simulink model "sampleModel1898"  (R2023a)
settings: Solver=VariableStepAuto  StartTime=0.0  StopTime=10.0  RelTol=1e-3
libraries: simulink x5, hdlsllib x3
settings Model: Creator=user1  LastModifiedBy=user1

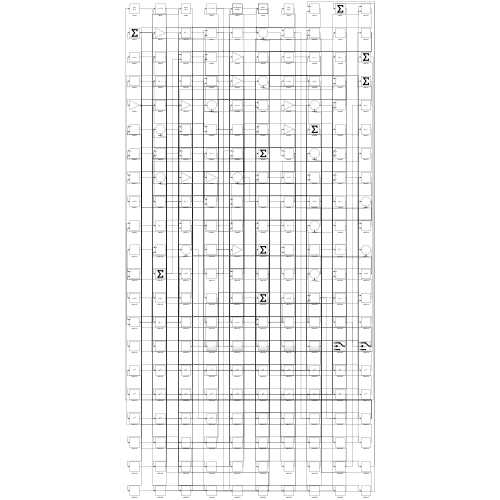
[thumbnail: Simulink's stored preview of the top-level diagram]
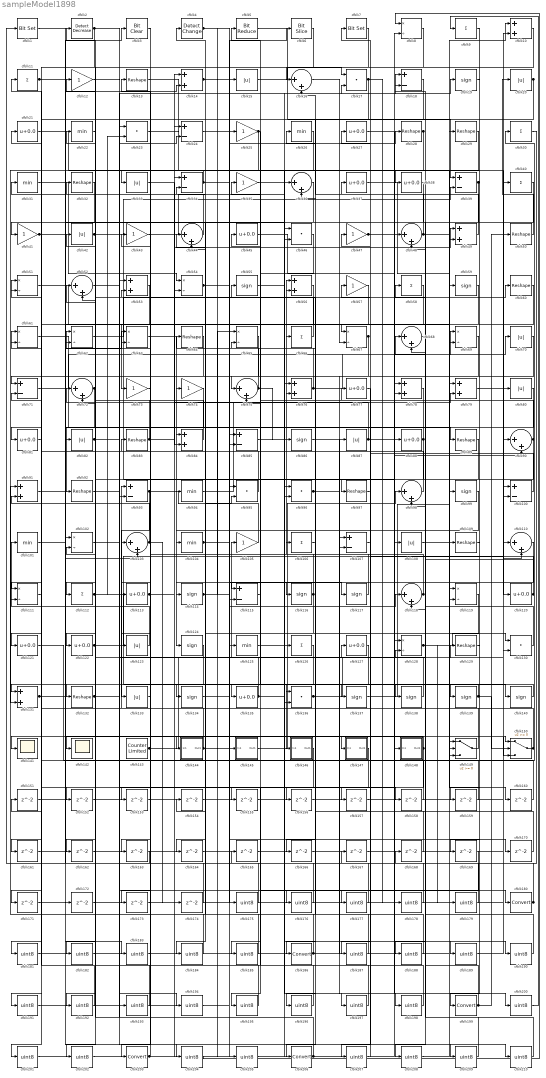
== system sampleModel1898 ==
  cfblk1 : simulink/Logic and Bit Operations/Bit Set  iBit=0
      settings: LibrarySourceBlock=|
      | hdlsllib/Logic and Bit
      | Operations/Bit Set
  cfblk{10,14,49,53,56,76,78..79,84,91,131} (11 alike) : Sum
  cfblk{18,24,34,39,71,85,93,100,107,115} (10 alike) : Sum  Inputs=+-
  cfblk{22,26,31,94,101,104,125} (7 alike) : MinMax
  cfblk{8,51,54,61..63,65,67,69,102,111,119,128} (13 alike) : Product  Inputs=*/  RndMeth=Zero  SaturateOnIntegerOverflow=on
  cfblk{16,36,44,48,52,68,72,75,90,98,103,110,118} (13 alike) : Sum  Inputs=|++
  cfblk{12,25,35,41,43,47,57,73..74,105} (10 alike) : Gain
  cfblk{9,11,30,40,58,66,106,112,126} (9 alike) : Sum  Inputs=+
  cfblk{15,20,33,42,70,80,82,87,108,123,133} (11 alike) : Abs  SaturateOnIntegerOverflow=off
  cfblk{13,28..29,32,50,60,64,83,89,92,97,109,129,132} (14 alike) : Reshape
  cfblk{21,27,37..38,45,77,81,88,113,120..122,127,135} (14 alike) : Bias  Bias=0.0  SaturateOnIntegerOverflow=off
  cfblk{19,55,59,86,99,114,116..117,124,134,137..140} (14 alike) : Signum
  cfblk{17,23,46,95..96,130,136} (7 alike) : DotProduct  OutDataTypeStr=Inherit: Inherit via internal rule
  cfblk141 : Scope
  cfblk142 : Scope
  cfblk143 : hdlsllib/Sources/Counter Limited  uplimit=7  tsamp=-1
  cfblk144 : Subsystem
      settings: LibrarySourceBlock=|
      | hdlsllib/Ports &
      | Subsystems/Subsystem
  cfblk145 : Subsystem
      settings: LibrarySourceBlock=|
      | hdlsllib/Ports &
      | Subsystems/Subsystem
  cfblk146 : Subsystem
      settings: LibrarySourceBlock=|
      | hdlsllib/Ports &
      | Subsystems/Subsystem
  cfblk147 : Subsystem
      settings: LibrarySourceBlock=|
      | hdlsllib/Ports &
      | Subsystems/Subsystem
  cfblk148 : Subsystem
      settings: LibrarySourceBlock=|
      | hdlsllib/Ports &
      | Subsystems/Subsystem
  cfblk149 : Switch  SaturateOnIntegerOverflow=off  InputSameDT=off
  cfblk150 : Switch  SaturateOnIntegerOverflow=off  InputSameDT=off
  cfblk{151..174} (24 alike) : Delay  SampleTime=1
  cfblk{175..179,181..185,187..198,200..202,204..205,207..210} (31 alike) : DataTypeConversion  OutDataTypeStr=uint8  SaturateOnIntegerOverflow=off  RndMeth=Floor
  cfblk{180,186,199,203,206} (5 alike) : DataTypeConversion  SaturateOnIntegerOverflow=off  RndMeth=Floor
  cfblk2 : simulink/Logic and Bit Operations/Detect Decrease  vinit=0.0  OutDataTypeStr=boolean
      settings: LibrarySourceBlock=|
      | hdlsllib/Logic and Bit
      | Operations/Detect
      | Decrease
  cfblk3 : simulink/Logic and Bit Operations/Bit Clear  iBit=0
      settings: LibrarySourceBlock=|
      | hdlsllib/Logic and Bit
      | Operations/Bit Clear
  cfblk4 : simulink/Logic and Bit Operations/Detect Change  vinit=0  OutDataTypeStr=boolean
      settings: LibrarySourceBlock=|
      | hdlsllib/Logic and Bit
      | Operations/Detect
      | Change
  cfblk5 : hdlsllib/Logic and Bit Operations/Bit Reduce  mode=AND
  cfblk6 : hdlsllib/Logic and Bit Operations/Bit Slice  lidx=7  ridx=0
  cfblk7 : simulink/Logic and Bit Operations/Bit Set  iBit=0
      settings: LibrarySourceBlock=|
      | hdlsllib/Logic and Bit
      | Operations/Bit Set
  wires:
  cfblk150/1 -> cfblk93/1, cfblk48/2
  cfblk49/1 -> cfblk26/1
  cfblk51/1 -> cfblk67/1
  cfblk39/1 -> cfblk81/1, cfblk164/1
  cfblk138/1 -> cfblk105/1
  cfblk139/1 -> cfblk132/1, cfblk150/2
  cfblk64/1 -> cfblk124/1
  cfblk5/1 -> cfblk39/1
  cfblk48/1 -> cfblk16/2, cfblk160/1
  cfblk31/1 -> cfblk54/1
  cfblk123/1 -> cfblk101/1
  cfblk15/1 -> cfblk17/1
  cfblk66/1 -> cfblk42/1
  cfblk93/1 -> cfblk133/1, cfblk95/2
  cfblk121/1 -> cfblk30/1
  cfblk16/1 -> cfblk67/2
  cfblk114/1 -> cfblk65/1, cfblk170/1
  cfblk72/1 -> cfblk92/1, cfblk182/1
  cfblk56/1 -> cfblk135/1
  cfblk67/1 -> cfblk161/1, cfblk162/1
  cfblk103/1 -> cfblk61/2, cfblk174/1
  cfblk131/1 -> cfblk3/1, cfblk63/1
  cfblk117/1 -> cfblk56/1
  cfblk111/1 -> cfblk11/1
  cfblk55/1 -> cfblk19/1
  cfblk62/1 -> cfblk60/1
  cfblk104/1 -> cfblk25/1, cfblk158/1
  cfblk50/1 -> cfblk20/1
  cfblk107/1 -> cfblk27/1
  cfblk145/1(Out1) -> cfblk98/1
  cfblk144/1(Out1) -> cfblk51/1, cfblk118/1
  cfblk70/1 -> cfblk107/2
  cfblk127/1 -> cfblk131/1
  cfblk13/1 -> cfblk100/1
  cfblk137/1 -> cfblk29/1
  cfblk133/1 -> cfblk13/1
  cfblk42/1 -> cfblk148/1(In1), cfblk39/2
  cfblk23/1 -> cfblk110/1
  cfblk83/1 -> cfblk2/1, cfblk79/2
  cfblk100/1 -> cfblk37/1
  cfblk17/1 -> cfblk121/1, cfblk178/1
  cfblk28/1 -> cfblk36/2, cfblk75/2
  cfblk32/1 -> cfblk41/1
  cfblk149/1 -> cfblk34/2
  cfblk20/1 -> cfblk103/1, cfblk93/2, cfblk196/1
  cfblk8/1 -> cfblk203/1
  cfblk115/1 -> cfblk45/1
  cfblk69/1 -> cfblk138/1
  cfblk63/1 -> cfblk84/1
  cfblk84/1 -> cfblk32/1
  cfblk2/1 -> cfblk71/1, cfblk54/2
  cfblk136/1 -> cfblk140/1, cfblk10/2
  cfblk21/1 -> cfblk109/1
  cfblk6/1 -> cfblk122/1
  cfblk36/1 -> cfblk112/1
  cfblk71/1 -> cfblk70/1
  cfblk82/1 -> cfblk155/1, cfblk156/1
  cfblk9/1 -> cfblk199/1
  cfblk34/1 -> cfblk28/1, cfblk33/1
  cfblk130/1 -> cfblk58/1
  cfblk58/1 -> cfblk78/2
  cfblk116/1 -> cfblk31/1, cfblk144/1(In1), cfblk136/2
  cfblk85/1 -> cfblk180/1
  cfblk46/1 -> cfblk75/1
  cfblk29/1 -> cfblk131/2
  cfblk112/1 -> cfblk146/1(In1), cfblk23/2
  cfblk98/1 -> cfblk61/1
  cfblk90/1 -> cfblk116/1, cfblk100/2, cfblk94/1, cfblk65/2
  cfblk60/1 -> cfblk73/1
  cfblk37/1 -> cfblk99/1
  cfblk118/1 -> cfblk114/1, cfblk62/1
  cfblk33/1 -> cfblk84/2
  cfblk78/1 -> cfblk97/1
  cfblk120/1 -> cfblk47/1, cfblk98/2
  cfblk105/1 -> cfblk64/1
  cfblk43/1 -> cfblk18/1
  cfblk76/1 -> cfblk69/1, cfblk4/1
  cfblk54/1 -> cfblk6/1, cfblk136/1
  cfblk25/1 -> cfblk115/1, cfblk115/2
  cfblk75/1 -> cfblk44/1, cfblk86/1
  cfblk94/1 -> cfblk48/1
  cfblk143/1 -> cfblk79/1, cfblk43/1
  cfblk44/1 -> cfblk12/1
  cfblk10/1 -> cfblk16/1
  cfblk95/1 -> cfblk21/1
  cfblk132/1 -> cfblk17/2, cfblk129/1
  cfblk14/1 -> cfblk117/1, cfblk145/1(In1)
  cfblk47/1 -> cfblk7/1, cfblk200/1
  cfblk135/1 -> cfblk76/1, cfblk62/2
  cfblk88/1 -> cfblk82/1, cfblk157/1
  cfblk53/1 -> cfblk111/1
  cfblk113/1 -> cfblk49/1, cfblk63/2
  cfblk24/1 -> cfblk38/1
  cfblk122/1 -> cfblk80/1, cfblk150/3
  cfblk4/1 -> cfblk137/1, cfblk205/1
  cfblk79/1 -> cfblk120/1
  cfblk148/1(Out1) -> cfblk141/1, cfblk191/1
  cfblk77/1 -> cfblk147/1(In1)
  cfblk57/1 -> cfblk206/1
  cfblk81/1 -> cfblk51/2
  cfblk45/1 -> cfblk88/1
  cfblk134/1 -> cfblk127/1
  cfblk41/1 -> cfblk150/1, cfblk46/2, cfblk89/1, cfblk181/1
  cfblk108/1 -> cfblk10/1
  cfblk59/1 -> cfblk113/1
  cfblk92/1 -> cfblk24/2
  cfblk26/1 -> cfblk96/2
  cfblk89/1 -> cfblk142/1
  cfblk96/1 -> cfblk66/1, cfblk189/1
  cfblk19/1 -> cfblk139/1
  cfblk140/1 -> cfblk134/1
  cfblk128/1 -> cfblk130/1, cfblk179/1
  cfblk106/1 -> cfblk186/1
  cfblk11/1 -> cfblk14/2, cfblk103/2, cfblk69/2
  cfblk99/1 -> cfblk104/1
  cfblk38/1 -> cfblk74/1
  cfblk27/1 -> cfblk90/2
  cfblk73/1 -> cfblk123/1
  cfblk87/1 -> cfblk149/2, cfblk72/1
  cfblk61/1 -> cfblk108/1
  cfblk151/1 -> cfblk128/1
  cfblk146/1(Out1) -> cfblk152/1
  cfblk124/1 -> cfblk153/1
  cfblk153/1 -> cfblk96/1
  cfblk155/1 -> cfblk78/1
  cfblk156/1 -> cfblk110/2
  cfblk157/1 -> cfblk49/2
  cfblk158/1 -> cfblk111/2
  cfblk109/1 -> cfblk159/1
  cfblk159/1 -> cfblk56/2
  cfblk160/1 -> cfblk34/1
  cfblk161/1 -> cfblk14/1
  cfblk162/1 -> cfblk130/2
  cfblk3/1 -> cfblk163/1
  cfblk163/1 -> cfblk1/1
  cfblk164/1 -> cfblk36/1
  cfblk165/1 -> cfblk149/3
  cfblk18/1 -> cfblk166/1
  cfblk166/1 -> cfblk119/1
  cfblk167/1 -> cfblk149/1
  cfblk30/1 -> cfblk168/1
  cfblk168/1 -> cfblk76/2
  cfblk129/1 -> cfblk169/1
  cfblk170/1 -> cfblk107/1
  cfblk65/1 -> cfblk171/1
  cfblk171/1 -> cfblk90/1
  cfblk101/1 -> cfblk172/1
  cfblk74/1 -> cfblk173/1
  cfblk173/1 -> cfblk53/2
  cfblk174/1 -> cfblk23/1
  cfblk154/1 -> cfblk175/1
  cfblk175/1 -> cfblk71/2
  cfblk80/1 -> cfblk176/1
  cfblk176/1 -> cfblk154/1
  cfblk102/1 -> cfblk177/1
  cfblk177/1 -> cfblk167/1
  cfblk178/1 -> cfblk102/1
  cfblk179/1 -> cfblk102/2
  cfblk180/1 -> cfblk165/1, cfblk77/1, cfblk18/2, cfblk5/1
  cfblk181/1 -> cfblk85/1
  cfblk182/1 -> cfblk85/2
  cfblk91/1 -> cfblk183/1
  cfblk183/1 -> cfblk87/1
  cfblk119/1 -> cfblk184/1
  cfblk184/1 -> cfblk91/1
  cfblk169/1 -> cfblk185/1
  cfblk185/1 -> cfblk91/2
  cfblk186/1 -> cfblk119/2, cfblk44/2
  cfblk97/1 -> cfblk187/1
  cfblk187/1 -> cfblk106/1
  cfblk40/1 -> cfblk188/1
  cfblk188/1 -> cfblk46/1
  cfblk189/1 -> cfblk40/1
  cfblk125/1 -> cfblk190/1
  cfblk190/1 -> cfblk128/2
  cfblk191/1 -> cfblk125/1
  cfblk22/1 -> cfblk192/1
  cfblk192/1 -> cfblk151/1
  cfblk12/1 -> cfblk193/1
  cfblk193/1 -> cfblk22/1
  cfblk52/1 -> cfblk194/1
  cfblk194/1 -> cfblk15/1
  cfblk147/1(Out1) -> cfblk195/1
  cfblk195/1 -> cfblk52/1
  cfblk196/1 -> cfblk52/2
  cfblk35/1 -> cfblk197/1
  cfblk197/1 -> cfblk55/1
  cfblk86/1 -> cfblk198/1
  cfblk198/1 -> cfblk35/1
  cfblk199/1 -> cfblk118/2, cfblk50/1
  cfblk200/1 -> cfblk9/1
  cfblk126/1 -> cfblk201/1
  cfblk201/1 -> cfblk24/1
  cfblk7/1 -> cfblk202/1
  cfblk202/1 -> cfblk126/1
  cfblk203/1 -> cfblk95/1, cfblk83/1
  cfblk172/1 -> cfblk204/1
  cfblk204/1 -> cfblk8/1
  cfblk205/1 -> cfblk8/2
  cfblk206/1 -> cfblk72/2, cfblk53/1
  cfblk110/1 -> cfblk207/1
  cfblk207/1 -> cfblk57/1
  cfblk68/1 -> cfblk208/1
  cfblk208/1 -> cfblk59/1
  cfblk1/1 -> cfblk209/1
  cfblk209/1 -> cfblk68/1
  cfblk152/1 -> cfblk210/1
  cfblk210/1 -> cfblk68/2

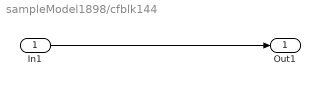
== system sampleModel1898/cfblk144 ==
  In1 : Inport
  Out1 : Outport
  wires:
  In1/1 -> Out1/1

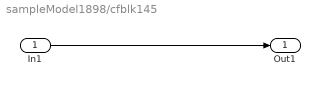
== system sampleModel1898/cfblk145 ==
  In1 : Inport
  Out1 : Outport
  wires:
  In1/1 -> Out1/1

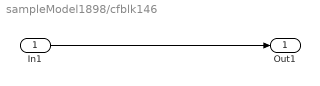
== system sampleModel1898/cfblk146 ==
  In1 : Inport
  Out1 : Outport
  wires:
  In1/1 -> Out1/1

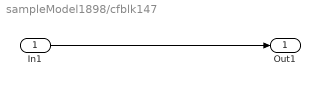
== system sampleModel1898/cfblk147 ==
  In1 : Inport
  Out1 : Outport
  wires:
  In1/1 -> Out1/1

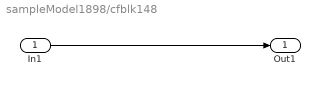
== system sampleModel1898/cfblk148 ==
  In1 : Inport
  Out1 : Outport
  wires:
  In1/1 -> Out1/1
